simulink model "HW2Part6"  (R2018a)
settings: Solver=FixedStepAuto  StartTime=0.0  StopTime=100  FixedStep=0.001  RelTol=1e-3
values from neighbouring files (symbols this model uses):
  A = M\APrime    [HW2.m]
  B = M\BPrime    [HW2.m]
  C = eye(4)    [HW2.m]
  Kq = 0.754    [HW2.m]
  Ktheta = -1.41    [HW2.m]
  x0 = [1;1;1;1]    [HW2.m]
settings Model: Creator=seongheonlee  LastModifiedBy=seongheonlee

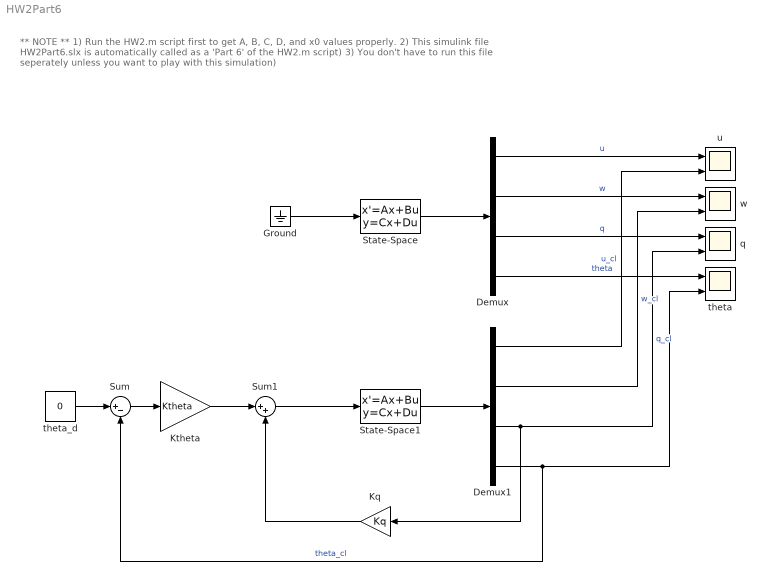
== system HW2Part6 ==
  note: ** NOTE **
      | 1) Run the HW2.m script first to get A, B, C, D, and x0 values properly.
      | 2) This simulink file HW2Part6.slx is automatically called as a 'Part 6' of the HW2.m script)
      | 3) You don't have to run this file seperately unless you want to play with this simulation)
  Demux : Demux
  Demux1 : Demux
  Ground : Ground
  Kq : Gain  Gain=Kq
  Ktheta : Gain  Gain=Ktheta
  State-Space : StateSpace  A=A  B=B  C=C  D=zeros(4,1)  InitialCondition=x0
  State-Space1 : StateSpace  A=A  B=B  C=C  D=zeros(4,1)  InitialCondition=x0
  Sum : Sum  Inputs=|+-
  Sum1 : Sum  Inputs=|++
  q : Scope  NumInputPorts=2
  theta : Scope  NumInputPorts=2
  theta_d : Constant  Value=0
  u : Scope  NumInputPorts=2
  w : Scope  NumInputPorts=2
  wires:
  State-Space/1 -> Demux/1
  Demux/1 -> u/1  "u"
  Demux/2 -> w/1  "w"
  Demux/3 -> q/1  "q"
  Demux/4 -> theta/1  "theta"
  State-Space1/1 -> Demux1/1
  Demux1/1 -> u/2  "u_cl"
  Demux1/2 -> w/2  "w_cl"
  Demux1/3 -> q/2, Kq/1  "q_cl"
  Demux1/4 -> theta/2, Sum/2  "theta_cl"
  theta_d/1 -> Sum/1
  Sum/1 -> Ktheta/1
  Ktheta/1 -> Sum1/1
  Kq/1 -> Sum1/2
  Sum1/1 -> State-Space1/1
  Ground/1 -> State-Space/1
